simulink model "Grid_Connected_PV_NG"  (R2020a)
settings: Solver=VariableStepAuto  StartTime=0.0  StopTime=10.0  RelTol=1e-3
values from neighbouring files (symbols this model uses):
  Cfmax = (0.05*Pmin)/(2*pi*f*U^2)    (= 5.51090523171e-06)    [filter_2.m]
  Lf = (0.1*U^2)/(2*pi*f*Pmin)    (= 0.00919278951299)    [filter_2.m]
  RLf = Lf*100    (= 0.919278951299)    [filter_2.m]
  Tss = 2.5e-6    (= 2.5e-06)    [filter_2.m]
libraries: powerlib x10, powerlib_meascontrol x4, simulink x2, re_lib x1
settings Model: Creator=Junaed  LastModifiedBy=Junaed

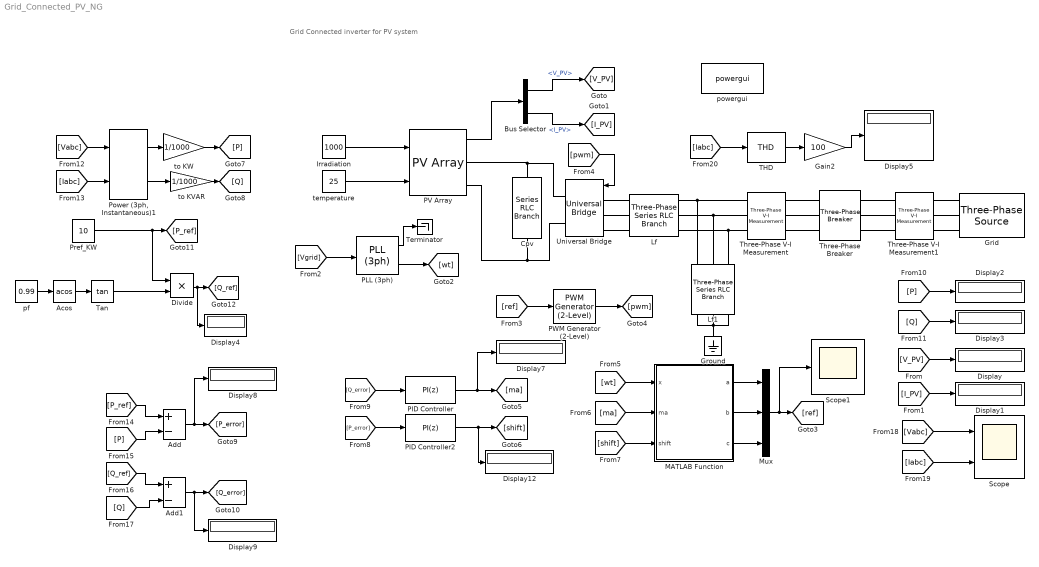
== system Grid_Connected_PV_NG ==
  note: Grid Connected inverter for PV system
  Acos : Trigonometry  Operator=acos
  Add : Sum  Inputs=+-
  Add1 : Sum  Inputs=+-
  Bus Selector : BusSelector  OutputSignals=V_PV,I_PV
  Cpv : powerlib/Elements/Series RLC Branch  LConnTagsString=__new0  RConnTagsString=__new0  BranchType=RC  Resistance=1e-3  Inductance=1000e-6  SetiL0=off  InitialCurrent=0  Capacitance=1000e-6  Setx0=off  InitialVoltage=0  Measurements=None
  Display{,1..5,7..9,12} (10 alike) : Display
  Divide : Product  Inputs=**
  Gain2 : Gain  Gain=100
  Grid : powerlib/Electrical Sources/Three-Phase Source  InternalConnection=Yg  VoltagePhases=off  Voltage=380  PhaseAngle=0  Voltage_phases=[25e3 25e3 25e3]/sqrt(3)  PhaseAngles_phases=[0 -120 +120]  Frequency=50  NonIdealSource=off  SpecifyImpedance=off  Resistance=0.8929  Inductance=16.58e-3  ShortCircuitLevel=100e6  BaseVoltage=380  XRratio=7  BusType=swing  Pref=10e3  Qref=0  Prefabc=[10e3, 10e3, 10e3]  Qrefabc=[0, 0, 0]  Qmin=-inf  Qmax=inf
  Ground : powerlib/Elements/Ground  LConnTagsString=a
  Irradiation : Constant  Value=1000
  Lf : powerlib/Elements/Three-Phase Series RLC Branch  LConnTagsString=A|B|C  RConnTagsString=A|B|C  BranchType=RL  Resistance=RLf  Inductance=Lf  Capacitance=1e-6  Measurements=None
  Lf1 : powerlib/Elements/Three-Phase Series RLC Branch  LConnTagsString=A|B|C  RConnTagsString=A|B|C  BranchType=RC  Resistance=RLf  Inductance=Lf  Capacitance=Cfmax  Measurements=None
  MATLAB Function : MATLAB Function  TreatAsAtomicUnit=on
  Mux : Mux  Inputs=3
  PID Controller : simulink/Continuous/PID Controller  Controller=PI  Form=Parallel  TimeDomain=Discrete-time  UseExternalTs=off  SampleTime=Tss*100  IntegratorMethod=Forward Euler  FilterMethod=Forward Euler  ControllerParametersSource=internal  P=0.01  I=1  D=0  UseFilter=on  N=100  TunerSelectOption=Transfer Function Based (PID Tuner App)  InitialConditionSource=internal  InitialConditionForIntegrator=0  InitialConditionForFilter=0  DifferentiatorICPrevScaledInput=0  ExternalReset=none  TrackingMode=off  Kt=1  LimitOutput=on  UpperSaturationLimit=1.1  LowerSaturationLimit=-1.1  LinearizeAsGain=on  AntiWindupMode=none  Kb=1  POutMin=[]  POutMax=[]  IOutMin=[]  IOutMax=[]  DOutMin=[]  DOutMax=[]  NOutMin=[]  NOutMax=[]  SumOutMin=[]  SumOutMax=[]  SaturationOutMin=[]  SaturationOutMax=[]  PParamMin=[]  PParamMax=[]  IParamMin=[]  IParamMax=[]  DParamMin=[]  DParamMax=[]  NParamMin=[]  NParamMax=[]  KbParamMin=[]  KbParamMax=[]  KtParamMin=[]  KtParamMax=[]  KbOutMin=[]  KbOutMax=[]  KtOutMin=[]  KtOutMax=[]  IntegratorOutMin=[]  IntegratorOutMax=[]  FilterOutMin=[]  FilterOutMax=[]  SumI1OutMin=[]  SumI1OutMax=[]  SumI2OutMin=[]  SumI2OutMax=[]  SumI3OutMin=[]  SumI3OutMax=[]  SumI4OutMin=[]  SumI4OutMax=[]  SumDOutMin=[]  SumDOutMax=[]  DifferentiatorOutMin=[]  DifferentiatorOutMax=[]  FilterDiffOutCoefMin=[]  FilterDiffOutCoefMax=[]  ReciprocalOutMin=[]  ReciprocalOutMax=[]  SumDenOutMin=[]  SumDenOutMax=[]  SumNumOutMin=[]  SumNumOutMax=[]  DivideOutMin=[]  DivideOutMax=[]  UdiffTsProdOutMin=[]  UdiffTsProdOutMax=[]  NTsProdOutMin=[]  NTsProdOutMax=[]  UintegralTsProdOutMin=[]  UintegralTsProdOutMax=[]  UngainTsProdOutMin=[]  UngainTsProdOutMax=[]  IntegratorContinuousStateAttributes=''  IntegratorStateMustResolveToSignalObject=off  IntegratorRTWStateStorageClass=Auto  FilterContinuousStateAttributes=''  FilterStateMustResolveToSignalObject=off  FilterRTWStateStorageClass=Auto  ParallelPVariant=InternalParameters  IdealPVariant=Disabled  IVariant=InternalParameters  DVariant=Disabled  IntegratorVariant=Discrete  SatVariant=Enabled  AWVariant=Passthrough  PCopyVariant=Disabled  TRVariant=Disabled  FdbkBlocksVariant=Forward  IdealPFdbkVariant=Disabled  SatFdbkVariant=Disabled  DerivativeFilterVariant=Disabled  NVariant=Disabled  NCopyVariant=Disabled_SignalSpec  FilterICVariant=Disabled  IntegratorICVariant=InternalICs  ExternalResetVariant=Disabled  TRSumVariant=Passthrough  SumFdbkVariant=Disabled  SumVariant=Sum_PI  TsampFilterVariant=InternalTs  TsampNgainVariant=Passthrough  TsampIntegralVariant=Passthrough
  PID Controller2 : simulink/Continuous/PID Controller  Controller=PI  Form=Parallel  TimeDomain=Discrete-time  UseExternalTs=off  SampleTime=Tss*100  IntegratorMethod=Forward Euler  FilterMethod=Forward Euler  ControllerParametersSource=internal  P=0.01  I=1  D=0  UseFilter=on  N=100  TunerSelectOption=Transfer Function Based (PID Tuner App)  InitialConditionSource=internal  InitialConditionForIntegrator=0  InitialConditionForFilter=0  DifferentiatorICPrevScaledInput=0  ExternalReset=none  TrackingMode=off  Kt=1  LimitOutput=on  UpperSaturationLimit=1.1  LowerSaturationLimit=-1.1  LinearizeAsGain=on  AntiWindupMode=none  Kb=1  POutMin=[]  POutMax=[]  IOutMin=[]  IOutMax=[]  DOutMin=[]  DOutMax=[]  NOutMin=[]  NOutMax=[]  SumOutMin=[]  SumOutMax=[]  SaturationOutMin=[]  SaturationOutMax=[]  PParamMin=[]  PParamMax=[]  IParamMin=[]  IParamMax=[]  DParamMin=[]  DParamMax=[]  NParamMin=[]  NParamMax=[]  KbParamMin=[]  KbParamMax=[]  KtParamMin=[]  KtParamMax=[]  KbOutMin=[]  KbOutMax=[]  KtOutMin=[]  KtOutMax=[]  IntegratorOutMin=[]  IntegratorOutMax=[]  FilterOutMin=[]  FilterOutMax=[]  SumI1OutMin=[]  SumI1OutMax=[]  SumI2OutMin=[]  SumI2OutMax=[]  SumI3OutMin=[]  SumI3OutMax=[]  SumI4OutMin=[]  SumI4OutMax=[]  SumDOutMin=[]  SumDOutMax=[]  DifferentiatorOutMin=[]  DifferentiatorOutMax=[]  FilterDiffOutCoefMin=[]  FilterDiffOutCoefMax=[]  ReciprocalOutMin=[]  ReciprocalOutMax=[]  SumDenOutMin=[]  SumDenOutMax=[]  SumNumOutMin=[]  SumNumOutMax=[]  DivideOutMin=[]  DivideOutMax=[]  UdiffTsProdOutMin=[]  UdiffTsProdOutMax=[]  NTsProdOutMin=[]  NTsProdOutMax=[]  UintegralTsProdOutMin=[]  UintegralTsProdOutMax=[]  UngainTsProdOutMin=[]  UngainTsProdOutMax=[]  IntegratorContinuousStateAttributes=''  IntegratorStateMustResolveToSignalObject=off  IntegratorRTWStateStorageClass=Auto  FilterContinuousStateAttributes=''  FilterStateMustResolveToSignalObject=off  FilterRTWStateStorageClass=Auto  ParallelPVariant=InternalParameters  IdealPVariant=Disabled  IVariant=InternalParameters  DVariant=Disabled  IntegratorVariant=Discrete  SatVariant=Enabled  AWVariant=Passthrough  PCopyVariant=Disabled  TRVariant=Disabled  FdbkBlocksVariant=Forward  IdealPFdbkVariant=Disabled  SatFdbkVariant=Disabled  DerivativeFilterVariant=Disabled  NVariant=Disabled  NCopyVariant=Disabled_SignalSpec  FilterICVariant=Disabled  IntegratorICVariant=InternalICs  ExternalResetVariant=Disabled  TRSumVariant=Passthrough  SumFdbkVariant=Disabled  SumVariant=Sum_PI  TsampFilterVariant=InternalTs  TsampNgainVariant=Passthrough  TsampIntegralVariant=Passthrough
  PLL (3ph) : powerlib_meascontrol/PLL/PLL (3ph)  Fmin=45  Par_Init=[0, 50]  ParK=[180, 3200, 1]  TcD=1e-4  MaxRateChangeFreq=12  FilterCutOffFreq=25  Ts=Tss  AGC=on
  PV Array : re_lib/Solar/PV Array  Npar=4  Nser=27  PlotType=array @ 1000 W/m2 & specified temperatures  S_vec="[ 1000  500  100 ]"  Temp_C_vec="[ 45 25  ]"  ModuleName=1Soltech 1STH-215-P  PlotWhenSelected=off  Pm=213.15  Ncell=60  Voc=36.3  Isc=7.84  Vm=29  Im=7.35  beta_Voc_pc=-0.36099  alpha_Isc_pc=0.102  beta_Voc=-0.13104  alpha_Isc=0.007997  IL=7.8649  I0=2.9259e-10  nI=0.98117  Rsh=313.3991  Rs=0.39383  RobustModel=off  RobustCellTemperature=25  BAL=on  Tc=1e-6  Tfilter=5e-5
  PWM Generator (2-Level) : powerlib_meascontrol/Pulse & Signal Generators/PWM Generator (2-Level)  ModulatorType=Three-phase bridge (6 pulses)  ModulatorMode=Unsynchronized  Fc=fsw  Pc=90  nF=27  MinMax="[ -1  1 ]"  SamplingTechnique=Natural  ModulatingSignals=off  m=0.8  Freq=60  Phase=0  Ts=Tss  ShowCarrierOutport=off
  "Power (3ph, Instantaneous)1" : powerlib_meascontrol/Measurements/Power (3ph, Instantaneous)
  Pref_KW : Constant  Value=10
  Scope : Scope  NumInputPorts=2
  Scope1 : Scope
  THD : powerlib_meascontrol/Measurements/THD  Freq=50  Ts=Tss
  Tan : Trigonometry  Operator=tan
  Terminator : Terminator
  Three-Phase V-I Measurement : powerlib/Measurements/Three-Phase V-I Measurement  VoltageMeasurement=phase-to-ground  SetLabelV=on  LabelV=Vabc  Vpu=off  VpuLL=off  CurrentMeasurement=yes  SetLabelI=on  LabelI=Iabc  Ipu=off  Pbase=100e6  Vbase=500e3  OutputType=Complex  PhasorSimulation=off  PSBequivalent=0
  Three-Phase V-I Measurement1 : powerlib/Measurements/Three-Phase V-I Measurement  VoltageMeasurement=phase-to-ground  SetLabelV=on  LabelV=Vgrid  Vpu=off  VpuLL=off  CurrentMeasurement=yes  SetLabelI=on  LabelI=Igrid  Ipu=off  Pbase=100e6  Vbase=500e3  OutputType=Complex  PhasorSimulation=off  PSBequivalent=0
  Three-Phase Breaker : powerlib/Elements/Three-Phase Breaker  InitialState=open  SwitchA=on  SwitchB=on  SwitchC=on  SwitchTimes="[1/50  10]"  External=off  BreakerResistance=0.01  SnubberResistance=1e6  SnubberCapacitance=inf  Measurements=None
  Universal Bridge : powerlib/Power Electronics/Universal Bridge  Arms=3  SnubberResistance=1e5  SnubberCapacitance=inf  Device=IGBT / Diodes  Ron=1e-3  Lon=0  ForwardVoltages="[  0  0  ]"  ForwardVoltage=0  GTOparameters=[ 10e-6 , 20e-6 ]  IGBTparameters=[ 1e-6 , 2e-6 ]  Measurements=None  Measurements_2=None  converterType=Rectifier
  pf : Constant  Value=0.99
  powergui : powerlib/powergui  Priority=1  SimulationMode=Discrete  SampleTime=Tss  frequency=60  Iterations=50  frequencyindice=50  Pbase=100e6  ErrMax=1e-4  UnitsV=kV  UnitsW=MW  buscounter=0  FunctionMessages=off  echomessages=off  EnableUseOfTLC=off  CurrentSourceSwitches=off  DisableSnubberDevices=off  DisableRonSwitches=off  DisableVfSwitches=off  DisplayEquations=off  AutomaticDiscreteSolvers=off  SolverType=Tustin/Backward Euler (TBE)  Interpol=off  ExternalGateDelay=off  methode=off  Ts=100  x0status=blocks  SPID=on  SwTol=0  HookPort=off  NonlinearTolerance=1e-4  nMaxIteration=100  ContinueOnMaxIteration=off  RestoreLinks=warning  ResistiveCurrentMeasurement=off  Frange=[0:2:500]  Ylog=off  Xlog=on  ShowGrid=off  save=off  variable=ZData  structure=0  ZoomFFT=off  StartTime=0.0  cycles=1  DisplayStyle=1  fundamental=60  FreqAxis=off  MaxFrequency=1000  frequencyindicesteady=1  RmsSteady=1  display=off
  temperature : Constant  Value=25
  to KVAR : Gain  Gain=1/1000
  to KW : Gain  Gain=1/1000
  wires:
  Irradiation/1 -> PV Array/1
  temperature/1 -> PV Array/2
  PV Array/1 -> Bus Selector/1
  Bus Selector/1 -> [V_PV]  "<V_PV>"
  Bus Selector/2 -> [I_PV]  "<I_PV>"
  [V_PV] -> Display/1
  [I_PV] -> Display1/1
  [Vgrid] -> PLL (3ph)/1
  PLL (3ph)/2 -> [wt]
  MATLAB Function/1(a) -> Mux/1
  MATLAB Function/2(b) -> Mux/2
  MATLAB Function/3(c) -> Mux/3
  Mux/1 -> Scope1/1, [ref]
  [ref] -> PWM Generator (2-Level)/1
  PWM Generator (2-Level)/1 -> [pwm]
  [pwm] -> Universal Bridge/1
  [wt] -> MATLAB Function/1(x)
  [ma] -> MATLAB Function/2(ma)
  [shift] -> MATLAB Function/3(shift)
  PID Controller/1 -> Display7/1, [ma]
  [Iabc] -> "Power (3ph, Instantaneous)1"/2
  [Vabc] -> "Power (3ph, Instantaneous)1"/1
  "Power (3ph, Instantaneous)1"/1 -> to KW/1
  "Power (3ph, Instantaneous)1"/2 -> to KVAR/1
  to KW/1 -> [P]
  to KVAR/1 -> [Q]
  [P] -> Display2/1
  [Q] -> Display3/1
  [P_ref] -> Add/1
  [P] -> Add/2
  Add/1 -> Display8/1, [P_error]
  Add1/1 -> Display9/1, [Q_error]
  [Q] -> Add1/2
  [Q_ref] -> Add1/1
  Pref_KW/1 -> [P_ref], Divide/1
  pf/1 -> Acos/1
  Acos/1 -> Tan/1
  Tan/1 -> Divide/2
  Divide/1 -> Display4/1, [Q_ref]
  [Vabc] -> Scope/1
  [Iabc] -> Scope/2
  [Iabc] -> THD/1
  THD/1 -> Gain2/1
  Gain2/1 -> Display5/1
  PID Controller2/1 -> Display12/1, [shift]
  [P_error] -> PID Controller2/1
  [Q_error] -> PID Controller/1
  PLL (3ph)/1 -> Terminator/1
  connections:
  PV Array/RConn1 -- Universal Bridge/RConn1 -- Cpv/LConn1
  PV Array/RConn2 -- Cpv/RConn1 -- Universal Bridge/RConn2
  Lf/LConn1 -- Universal Bridge/LConn1
  Universal Bridge/LConn2 -- Lf/LConn2
  Universal Bridge/LConn3 -- Lf/LConn3
  Lf/RConn1 -- Lf1/LConn1 -- Three-Phase V-I Measurement/LConn1
  Lf/RConn2 -- Lf1/LConn2 -- Three-Phase V-I Measurement/LConn2
  Lf/RConn3 -- Lf1/LConn3 -- Three-Phase V-I Measurement/LConn3
  Three-Phase Breaker/LConn1 -- Three-Phase V-I Measurement/RConn1
  Three-Phase Breaker/LConn2 -- Three-Phase V-I Measurement/RConn2
  Three-Phase Breaker/LConn3 -- Three-Phase V-I Measurement/RConn3
  Three-Phase Breaker/RConn1 -- Three-Phase V-I Measurement1/RConn1
  Three-Phase Breaker/RConn2 -- Three-Phase V-I Measurement1/RConn2
  Three-Phase Breaker/RConn3 -- Three-Phase V-I Measurement1/RConn3
  Three-Phase V-I Measurement1/LConn1 -- Grid/RConn1
  Three-Phase V-I Measurement1/LConn2 -- Grid/RConn2
  Three-Phase V-I Measurement1/LConn3 -- Grid/RConn3
  Lf1/RConn1 -- Ground/LConn1 -- Lf1/RConn3 -- Lf1/RConn2

== matlab function Grid_Connected_PV_NG/MATLAB Function ==
  data: x input; a output; ma input; shift input; b output; c output
function [a,b,c] = ref_generator(x,ma,shift)
    
a = (ma * ( sin((x) +shift)));
b = (ma * (sin((x)+shift - (2*pi/3))));
c = (ma * (sin((x)+shift + (2*pi/3))));

end

% ma is modulation index
% x is wt rad/s
%shift_k is phase shift angle rad
